simulink model "Block_diagram"  (R2018a)
settings: Solver=VariableStepAuto  StartTime=0.0  StopTime=10.0  RelTol=1e-3
libraries: simulink x3, arduinolib x3
settings Model: Creator=adiravishankara  LastModifiedBy=adiravishankara

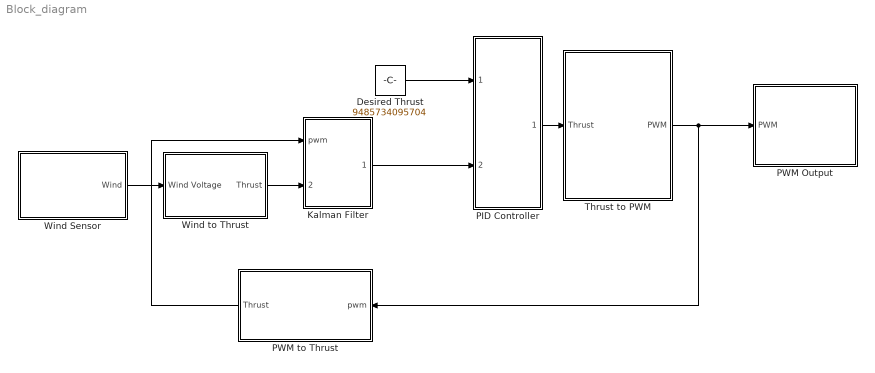
== system Block_diagram ==
  "Desired Thrust " : Constant  Value=9485734095704
  Kalman Filter : Subsystem
  PID Controller : Subsystem
  "PWM Output " : Subsystem
  PWM to Thrust : Subsystem
  Thrust to PWM : Subsystem
  Wind Sensor : Subsystem
  Wind to Thrust : Subsystem
  wires:
  Wind Sensor/1(Wind) -> Wind to Thrust/1(Wind Voltage)
  Thrust to PWM/1(PWM) -> PWM to Thrust/1(pwm), "PWM Output "/1(PWM)
  PWM to Thrust/1(Thrust) -> Kalman Filter/1(pwm)
  Wind to Thrust/1(Thrust) -> Kalman Filter/2(Wind_thrust)
  Kalman Filter/1(Wind estimate) -> PID Controller/2(Actual Thrust)
  "Desired Thrust "/1 -> PID Controller/1(Thrust Desired)
  PID Controller/1("Thrust ") -> Thrust to PWM/1(Thrust)

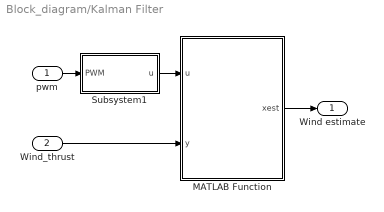
== system Block_diagram/Kalman Filter ==
  pwm : Inport
  Wind_thrust : Inport  Port=2
  MATLAB Function : MATLAB Function  TreatAsAtomicUnit=on
  Subsystem1 : Subsystem
  Wind estimate : Outport
  wires:
  Subsystem1/1(u) -> MATLAB Function/1(u)
  Wind_thrust/1 -> MATLAB Function/2(y)
  pwm/1 -> Subsystem1/1(PWM)
  MATLAB Function/1(xest) -> Wind estimate/1

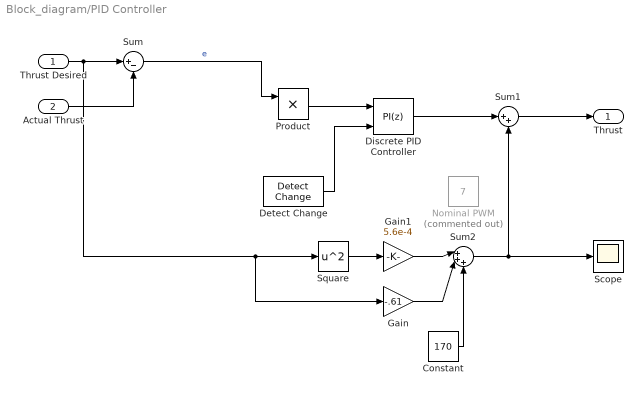
== system Block_diagram/PID Controller ==
  Thrust Desired : Inport
  Actual Thrust : Inport  Port=2
  Constant : Constant  Value=170
  Detect Change : simulink/Logic and Bit Operations/Detect Change  vinit=0  OutDataTypeStr=boolean
  Discrete PID Controller : simulink/Continuous/PID Controller  Controller=PI  TimeDomain=Discrete-time  SampleTime=0.01  IntegratorMethod=Forward Euler  FilterMethod=Forward Euler  Form=Parallel  UseFilter=on  ControllerParametersSource=internal  P=0.05  I=0.01  D=0  N=100  InitialConditionSource=internal  InitialConditionForIntegrator=0  InitialConditionForFilter=0  ExternalReset=rising  LimitOutput=off  UpperSaturationLimit=inf  LowerSaturationLimit=-inf  LinearizeAsGain=off  AntiWindupMode=none  Kb=1  TrackingMode=off  Kt=1  PParamMin=[]  PParamMax=[]  IParamMin=[]  IParamMax=[]  DParamMin=[]  DParamMax=[]  NParamMin=[]  NParamMax=[]  KbParamMin=[]  KbParamMax=[]  KtParamMin=[]  KtParamMax=[]  POutMin=[]  POutMax=[]  IOutMin=[]  IOutMax=[]  DOutMin=[]  DOutMax=[]  NOutMin=[]  NOutMax=[]  KbOutMin=[]  KbOutMax=[]  KtOutMin=[]  KtOutMax=[]  IntegratorOutMin=[]  IntegratorOutMax=[]  FilterOutMin=[]  FilterOutMax=[]  SumOutMin=[]  SumOutMax=[]  SumI1OutMin=[]  SumI1OutMax=[]  SumI2OutMin=[]  SumI2OutMax=[]  SumI3OutMin=[]  SumI3OutMax=[]  SumDOutMin=[]  SumDOutMax=[]  SaturationOutMin=[]  SaturationOutMax=[]  IntegratorContinuousStateAttributes=''  IntegratorStateMustResolveToSignalObject=off  IntegratorRTWStateStorageClass=Auto  FilterContinuousStateAttributes=''  FilterStateMustResolveToSignalObject=off  FilterRTWStateStorageClass=Auto  DifferentiatorICPrevScaledInput=0  DifferentiatorOutMin=[]  DifferentiatorOutMax=[]  FilterDiffOutCoefMin=[]  FilterDiffOutCoefMax=[]  SumDenOutMin=[]  SumDenOutMax=[]  SumNumOutMin=[]  SumNumOutMax=[]  ReciprocalOutMin=[]  ReciprocalOutMax=[]  DivideOutMin=[]  DivideOutMax=[]  TunerSelectOption=Transfer Function Based (PID Tuner App)
  Gain : Gain  Gain=-.61
  Gain1 : Gain  Gain=5.6e-4
  Nominal PWM : Constant  Commented=on  Value=7  SampleTime=0.01
  Product : Product
  Scope : Scope
  Square : Math  Operator=square  SaturateOnIntegerOverflow=on
  Sum : Sum  Inputs=|+-
  Sum1 : Sum  Inputs=|++
  Sum2 : Sum  Inputs=|+++
  "Thrust " : Outport
  wires:
  Detect Change/1 -> Discrete PID Controller/2
  Thrust Desired/1 -> Gain/1, Square/1, Sum/1
  Discrete PID Controller/1 -> Sum1/1
  Sum/1 -> Product/1  "e"
  Actual Thrust/1 -> Sum/2
  Sum1/1 -> "Thrust "/1
  Product/1 -> Discrete PID Controller/1
  Gain/1 -> Sum2/2
  Gain1/1 -> Sum2/1
  Constant/1 -> Sum2/3
  Square/1 -> Gain1/1
  Sum2/1 -> Sum1/2, Scope/1

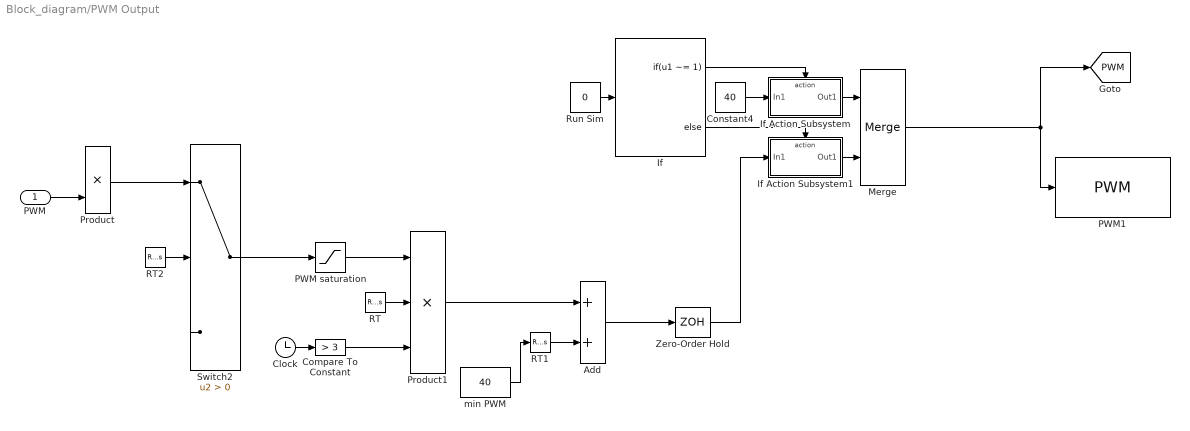
== system Block_diagram/PWM Output  ==
  PWM : Inport
  Add : Sum
  Clock : Clock
      settings: Decimation=2
  Compare To Constant : simulink/Logic and Bit Operations/Compare To Constant  relop=>  const=3  OutDataTypeStr=boolean
  Constant4 : Constant  Value=40  SampleTime=0.01
  If : If  IfExpression=u1 ~= 1
  If Action Subsystem : Subsystem  TreatAsAtomicUnit=on
  If Action Subsystem1 : Subsystem  TreatAsAtomicUnit=on
  Merge : Merge
  PWM saturation : Saturate  UpperLimit=40  LowerLimit=0
  PWM1 : arduinolib/PWM  pinNumber=12  EnableInputFrequency=off  InitialFrequency=2000  InitialDutyCycle=0  NotificationType=None  blockPlatform=arduino
  Product : Product
  Product1 : Product  Inputs=3
  RT : RateTransition  OutPortSampleTime=0.01
  RT1 : RateTransition  OutPortSampleTime=0.01
  RT2 : RateTransition  OutPortSampleTime=0.01
  Run Sim : Constant  Value=0  SampleTime=0.01
  Switch2 : Switch  Criteria=u2 > Threshold
  Zero-Order Hold : ZeroOrderHold  SampleTime=0.01
  min PWM : Constant  Value=40  SampleTime=0.01
  tag scope: PWM=global
  wires:
  Clock/1 -> Compare To Constant/1
  min PWM/1 -> RT1/1
  Compare To Constant/1 -> Product1/3
  ? -> RT2/1
  ? -> Switch2/3
  PWM/1 -> Product/2
  Switch2/1 -> PWM saturation/1
  ? -> RT/1
  Product1/1 -> Add/1
  PWM saturation/1 -> Product1/1
  Product/1 -> Switch2/1
  ? -> Product/1
  If/1 -> If Action Subsystem/Action
  Run Sim/1 -> If/1
  Constant4/1 -> If Action Subsystem/1(In1)
  Add/1 -> Zero-Order Hold/1
  If/2 -> If Action Subsystem1/Action
  If Action Subsystem1/1(Out1) -> Merge/2
  Merge/1 -> [PWM], PWM1/1
  Zero-Order Hold/1 -> If Action Subsystem1/1(In1)
  RT/1 -> Product1/2
  RT1/1 -> Add/2
  RT2/1 -> Switch2/2
  If Action Subsystem/1(Out1) -> Merge/1

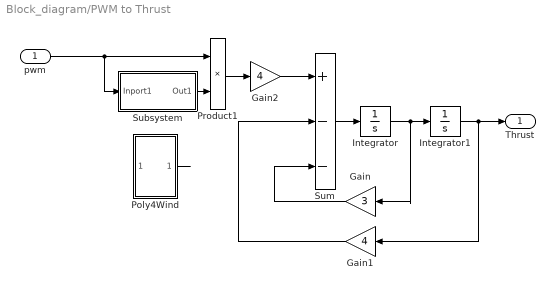
== system Block_diagram/PWM to Thrust ==
  pwm : Inport
  Gain : Gain  Gain=3
  Gain1 : Gain  Gain=4
  Gain2 : Gain  Gain=4
  Integrator : Integrator
  Integrator1 : Integrator
  "Poly4Wind " : Subsystem
  Product1 : Product
  Subsystem : Subsystem
  Sum : Sum  Inputs=+--
  Thrust : Outport
  wires:
  Product1/1 -> Gain2/1
  Integrator/1 -> Gain/1, Integrator1/1
  Sum/1 -> Integrator/1
  Integrator1/1 -> Gain1/1, Thrust/1
  Gain/1 -> Sum/3
  Gain1/1 -> Sum/2
  Gain2/1 -> Sum/1
  "Poly4Wind "/1(Out1) -> ?
  pwm/1 -> Subsystem/1(Inport1), Product1/1
  Subsystem/1(Out1) -> Product1/2

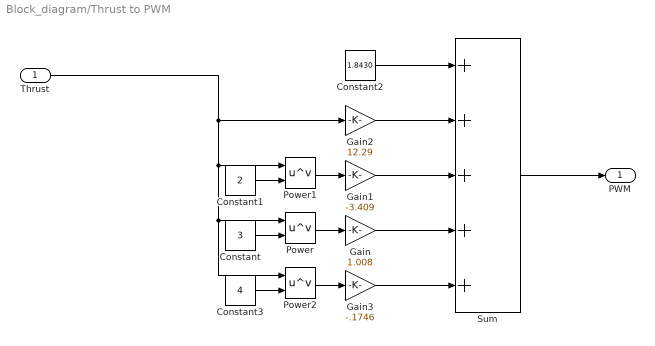
== system Block_diagram/Thrust to PWM ==
  Thrust : Inport
  Constant : Constant  Value=3
  Constant1 : Constant  Value=2
  Constant2 : Constant  Value=1.8430
  Constant3 : Constant  Value=4
  Gain : Gain  Gain=1.008
  Gain1 : Gain  Gain=-3.409
  Gain2 : Gain  Gain=12.29
  Gain3 : Gain  Gain=-.1746
  Power : Math  Operator=pow  SaturateOnIntegerOverflow=on
  Power1 : Math  Operator=pow  SaturateOnIntegerOverflow=on
  Power2 : Math  Operator=pow  SaturateOnIntegerOverflow=on
  Sum : Sum  Inputs=+++++
  PWM : Outport
  wires:
  Gain/1 -> Sum/4
  Power/1 -> Gain/1
  Power1/1 -> Gain1/1
  Thrust/1 -> Power2/1, Power/1, Power1/1, Gain2/1
  Gain1/1 -> Sum/3
  Constant/1 -> Power/2
  Sum/1 -> PWM/1
  Gain2/1 -> Sum/2
  Constant1/1 -> Power1/2
  Constant2/1 -> Sum/1
  Constant3/1 -> Power2/2
  Power2/1 -> Gain3/1
  Gain3/1 -> Sum/5

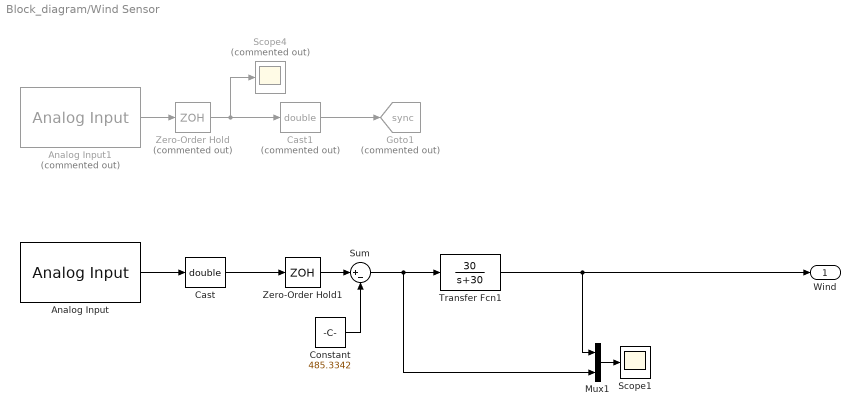
== system Block_diagram/Wind Sensor ==
  Analog Input : arduinolib/Analog Input  pinNumber=2  ReadResultsOnly=off  ConversionTriggerSource=Software  ExternalTriggerType=uint32(0)  OutputDataType=uint16  EnableConversionCompleteNotify=off  EnableOuputStatus=off  SampleTime=0.01  blockPlatform=arduino
  Analog Input1 : arduinolib/Analog Input  Commented=on  pinNumber=3  ReadResultsOnly=off  ConversionTriggerSource=Software  ExternalTriggerType=uint32(0)  OutputDataType=uint16  EnableConversionCompleteNotify=off  EnableOuputStatus=off  SampleTime=0.01  blockPlatform=arduino
  Cast : DataTypeConversion  OutDataTypeStr=double
  Cast1 : DataTypeConversion  Commented=on  OutDataTypeStr=double
  Constant : Constant  Value=485.3342
  Goto1 : Goto  Commented=on  GotoTag=sync  TagVisibility=global
  Mux1 : Mux  Inputs=2
  Scope1 : Scope
  Scope4 : Scope  Commented=on
  Sum : Sum  Inputs=|+-
  Transfer Fcn1 : TransferFcn  Numerator=[30]  Denominator=[1 30]
  Zero-Order Hold : ZeroOrderHold  Commented=on  SampleTime=0.01
  Zero-Order Hold1 : ZeroOrderHold  SampleTime=0.01
  Wind : Outport
  wires:
  Zero-Order Hold/1 -> Cast1/1, Scope4/1
  Analog Input/1 -> Cast/1
  Cast/1 -> Zero-Order Hold1/1
  Analog Input1/1 -> Zero-Order Hold/1
  Cast1/1 -> Goto1/1
  Zero-Order Hold1/1 -> Sum/1
  Transfer Fcn1/1 -> Mux1/1, Wind/1
  Mux1/1 -> Scope1/1
  Constant/1 -> Sum/2
  Sum/1 -> Mux1/2, Transfer Fcn1/1

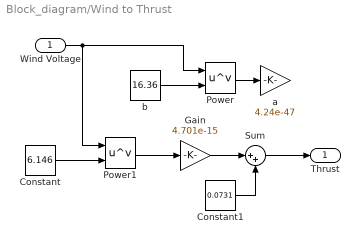
== system Block_diagram/Wind to Thrust ==
  Wind Voltage : Inport
  Constant : Constant  Value=6.146
  Constant1 : Constant  Value=0.0731
  Gain : Gain  Gain=4.701e-15
  Power : Math  Operator=pow  SaturateOnIntegerOverflow=on
  Power1 : Math  Operator=pow  SaturateOnIntegerOverflow=on
  Sum : Sum  Inputs=|++
  a : Gain  Gain=4.24e-47
  b : Constant  Value=16.36
  Thrust : Outport
  wires:
  b/1 -> Power/2
  Power/1 -> a/1
  Wind Voltage/1 -> Power1/1, Power/1
  Constant/1 -> Power1/2
  Power1/1 -> Gain/1
  Gain/1 -> Sum/1
  Constant1/1 -> Sum/2
  Sum/1 -> Thrust/1

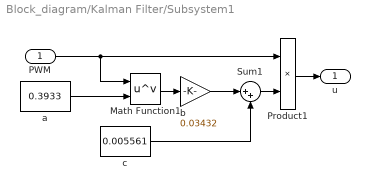
== system Block_diagram/Kalman Filter/Subsystem1 ==
  PWM : Inport
  Math Function1 : Math  Operator=pow  SaturateOnIntegerOverflow=on
  Product1 : Product
  Sum1 : Sum  Inputs=|++
  a : Constant  Value=0.3933
  b : Gain  Gain=0.03432
  c : Constant  Value=0.005561
  u : Outport
  wires:
  Sum1/1 -> Product1/2
  Product1/1 -> u/1
  a/1 -> Math Function1/2
  b/1 -> Sum1/1
  PWM/1 -> Math Function1/1, Product1/1
  Math Function1/1 -> b/1
  c/1 -> Sum1/2

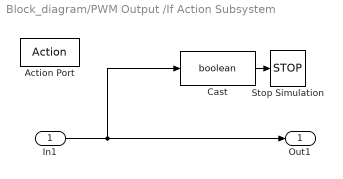
== system Block_diagram/PWM Output /If Action Subsystem ==
  In1 : Inport
  Action Port : ActionPort
  Cast : DataTypeConversion  OutDataTypeStr=boolean
  Stop Simulation : Stop
  Out1 : Outport
  wires:
  In1/1 -> Cast/1, Out1/1
  Cast/1 -> Stop Simulation/1

== system Block_diagram/PWM Output /If Action Subsystem1 ==
  In1 : Inport
  Action Port : ActionPort
  Out1 : Outport
  wires:
  In1/1 -> Out1/1

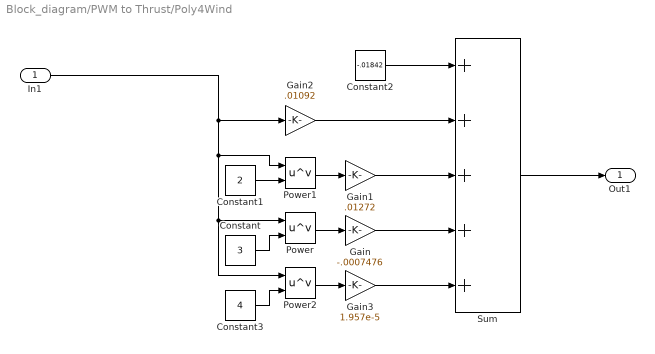
== system Block_diagram/PWM to Thrust/Poly4Wind  ==
  In1 : Inport
  Constant : Constant  Value=3
  Constant1 : Constant  Value=2
  Constant2 : Constant  Value=-.01842
  Constant3 : Constant  Value=4
  Gain : Gain  Gain=-.0007476
  Gain1 : Gain  Gain=.01272
  Gain2 : Gain  Gain=.01092
  Gain3 : Gain  Gain=1.957e-5
  Power : Math  Operator=pow  SaturateOnIntegerOverflow=on
  Power1 : Math  Operator=pow  SaturateOnIntegerOverflow=on
  Power2 : Math  Operator=pow  SaturateOnIntegerOverflow=on
  Sum : Sum  Inputs=+++++
  Out1 : Outport
  wires:
  Gain/1 -> Sum/4
  Power/1 -> Gain/1
  Power1/1 -> Gain1/1
  In1/1 -> Power2/1, Power/1, Power1/1, Gain2/1
  Gain1/1 -> Sum/3
  Constant/1 -> Power/2
  Sum/1 -> Out1/1
  Gain2/1 -> Sum/2
  Constant1/1 -> Power1/2
  Constant2/1 -> Sum/1
  Constant3/1 -> Power2/2
  Power2/1 -> Gain3/1
  Gain3/1 -> Sum/5

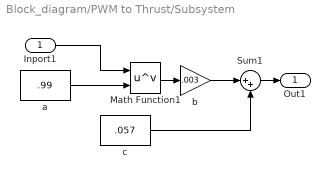
== system Block_diagram/PWM to Thrust/Subsystem ==
  Inport1 : Inport
  Math Function1 : Math  Operator=pow  SaturateOnIntegerOverflow=on
  Sum1 : Sum  Inputs=|++
  a : Constant  Value=.99
  b : Gain  Gain=.003
  c : Constant  Value=.057
  Out1 : Outport
  wires:
  a/1 -> Math Function1/2
  b/1 -> Sum1/1
  Inport1/1 -> Math Function1/1
  Math Function1/1 -> b/1
  Sum1/1 -> Out1/1
  c/1 -> Sum1/2

== matlab function Block_diagram/Kalman Filter/MATLAB Function ==
  settings: updateMethod=DISCRETE
  data: u input; xest output; y input
function xest  = fcn(u, y)
persistent P xh
if isempty(P)
    P = eye(2);
    xh = zeros(2,1);
end
% A = [0 1; -4 -3];
% B = [0; 4];
% C = [1 0];

Ad = [0.9998  0.009851; -0.0394    0.9702];
Bd = [0.000198; 0.0394];
Cd = [1 0];

Q = 1;
R = diag([5,5]);


% Model information
xh_bar = Ad * xh + Bd * u;
P_bar = Ad * P * Ad' + R;

% Measurement update
K = P_bar * Cd' * (Cd * P_bar * Cd' + Q)^-1;
xh = xh_bar + K * (y - Cd * xh_bar);
P = (1 - K * Cd) * P_bar;

xest = xh;
